simulink model "ssc_bridge_rectifier_rt"  (R2015b)
settings: Solver=ode3  StartTime=0.0  StopTime=0.05  FixedStep=Ts  MaxStep=0.001  RelTol=1e-3
PostLoadFcn:
  | Ts=100e-6;
InitFcn:
  | Ts=100e-6;
undefined symbols (not defined in the file): another_event_name, my_event_name
libraries: fl_lib x11, opal_lib x4, rtlab x3, nesl_utility x3
Description:
  | Full-Wave Bridge Rectifier
  | 
  | This is a model of a power supply that converts 120 volts AC to 12  volts DC. The
  | transformer has a turns ratio of 14, stepping the supply down to 8.6 volts rms, i.e.
  | 8.6*sqrt(2) = 12 volts pk-pk. The full-wave bridge rectifier plus capacitor combination
  | then converts this to DC. The resistor represents a typical load.
  | 
  | The model can be used to size the capacitor required for a specified load.  For a
  | given size of capacitor, as the load resistance is increased, the ripple on the DC
  | voltage increases. The model can also be used to drive an application circuit in
  | order to assess the effect of the ripple.
  | 
  | 
  | Copyright 2008 The MathWorks(TM), Inc.
settings Model: ExtModeAutoUpdateStatusClock=off  Creator=rhyde  LastModifiedBy=NesrineBradai
settings DataIOCC: SaveFormat=Array  SignalLoggingSaveFormat=ModelDataLogs  SaveOutput=off  SignalLogging=off  SaveTime=off
settings OptimizationCC: BlockReduction=off  OptimizeBlockIOStorage=off  BufferReuse=off  ExpressionFolding=off  ExpressionDepthLimit=2147483647  LocalBlockOutputs=off  InitFltsAndDblsToZero=on
settings DebuggingCC: SaveWithParameterizedLinksMsg=none  UnderspecifiedInitializationDetection=Classic  MergeDetectMultiDrivingBlocksExec=none  SignalResolutionControl=TryResolveAllWithWarning  SolverPrmCheckMsg=warning  FcnCallInpInsideContextMsg=EnableAllAsWarning  AllowSymbolicDim=on  StateNameClashWarn=warning
settings HardwareCC: ProdBitPerPointer=32  ProdLargestAtomicFloat=None  ProdIntDivRoundTo=Undefined  ProdEndianess=Unspecified  ProdWordSize=32  ProdHWDeviceType=32-bit Generic
settings GRTTargetCC: TargetFcnLib=ansi_tfl_tmw.mat  CombineOutputUpdateFcns=off  GRTInterface=on
settings ConfigComp: CovModelRefEnable=Off
settings SimscapeCC: SimscapeNormalizeSystem=off

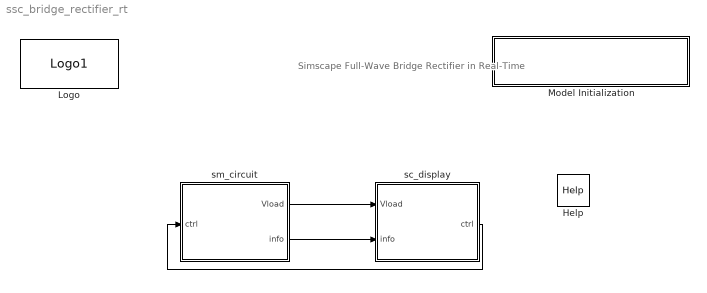
== system ssc_bridge_rectifier_rt ==
  note: Simscape Full-Wave Bridge Rectifier in Real-Time
  Help : opal_lib/Help  docfile=../../help/help.html
  Logo : opal_lib/Logo1  vide=[]
  Model Initialization : Subsystem  mask(Model Functions){InitFcnX=Ts=100e-6;, prel=off, posl=on, inif=on, strf=off}
      mask prompts: InitFcnX "Initialisation"; prel "Preload Function"; posl "PostLoad Function"; inif "InitFcn"; strf "StartFcn"
      mask init:
      | currentBlock = gcb;
      | root = bdroot(currentBlock);
      | 
      | if ~strcmp(get_param(root,'BlockDiagramType'),'library')
      |     if prel==1
      |         set_param(root, 'PreLoadFcn', InitFcnX);
      |     else
      |         set_param(root, 'PreLoadFcn', '');
      |     end
      |     if inif==1
      |         set_param(root, 'InitFcn', InitFcnX);
      |     else
      |         set_param(root, 'InitFcn', '');
      |     end
      |     if strf==1
      |         set_param(root, 'StartFcn', InitFcnX);
      |     else
      |         set_param(root, 'StartFcn', '');
      |     end
      |     if posl==1
      |         set_param(root, 'PostLoadFcn', InitFcnX);
      |     else
      |         set_param(root, 'PostLoadFcn', '');
      |     end
      | end
      | 
      | pos = get_param(currentBlock, 'Position');
      | width = pos(3) - pos(1); height = pos(4) - pos(2);
      | txt = [ upper(root) '\n' '- InitFcn. . . . . '  get_param(root, 'InitFcn') ];
      settings: CopyFcn=set_param(gcb,'LinkStatus','none')
      mask Display: text(5, height*0.5, txt, 'horizontalAlignment', 'left', 'verticalAlignment', 'middle') ;
  sc_display : Subsystem
  sm_circuit : Subsystem
  wires:
  sm_circuit/1(Vload) -> sc_display/1(Vload)
  sm_circuit/2(info) -> sc_display/2(info)
  sc_display/1(ctrl) -> sm_circuit/1(ctrl)

== system ssc_bridge_rectifier_rt/Model Initialization ==

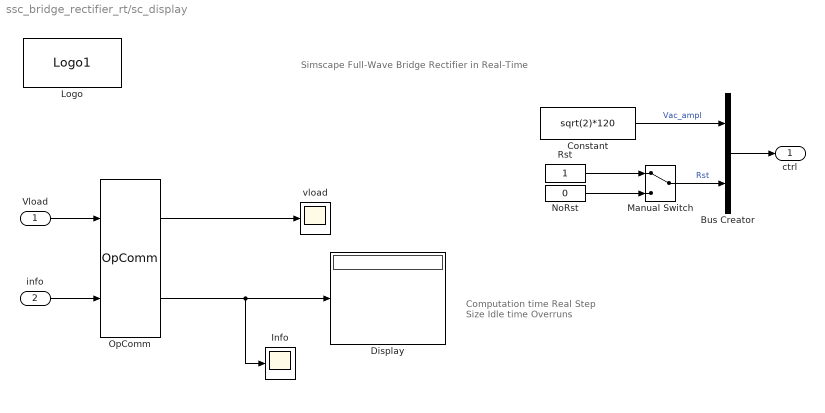
== system ssc_bridge_rectifier_rt/sc_display ==
  note: Computation time
      | Real Step Size
      | Idle time
      | Overruns
  note: Simscape Full-Wave Bridge Rectifier in Real-Time
  Vload : Inport
  info : Inport  Port=2
  Bus Creator : BusCreator  Inputs=2
  Constant : Constant  Value=sqrt(2)*120
  Display : Display
  Info : Scope
  Logo : opal_lib/Logo1  vide=[]
  Manual Switch : ManualSwitch
  NoRst : Constant  Value=0
  OpComm : rtlab/OpComm  nbport=2  groupe_acq=1  subsys_rate=0  st=0  Synchronization=on  Interpolation=on  Threshold=1.0  Missed_Data=off  Sim_Time=off  Samples=off  dynSigOut=off  from_console=0  warning_done=off  writeOpCommFile=off  Offset=off
  Rst : Constant
  vload : Scope
  ctrl : Outport
  wires:
  Vload/1 -> OpComm/1
  OpComm/1 -> vload/1
  info/1 -> OpComm/2
  OpComm/2 -> Info/1, Display/1
  Rst/1 -> Manual Switch/1
  NoRst/1 -> Manual Switch/2
  Bus Creator/1 -> ctrl/1
  Constant/1 -> Bus Creator/1  "Vac_ampl"
  Manual Switch/1 -> Bus Creator/2  "Rst"

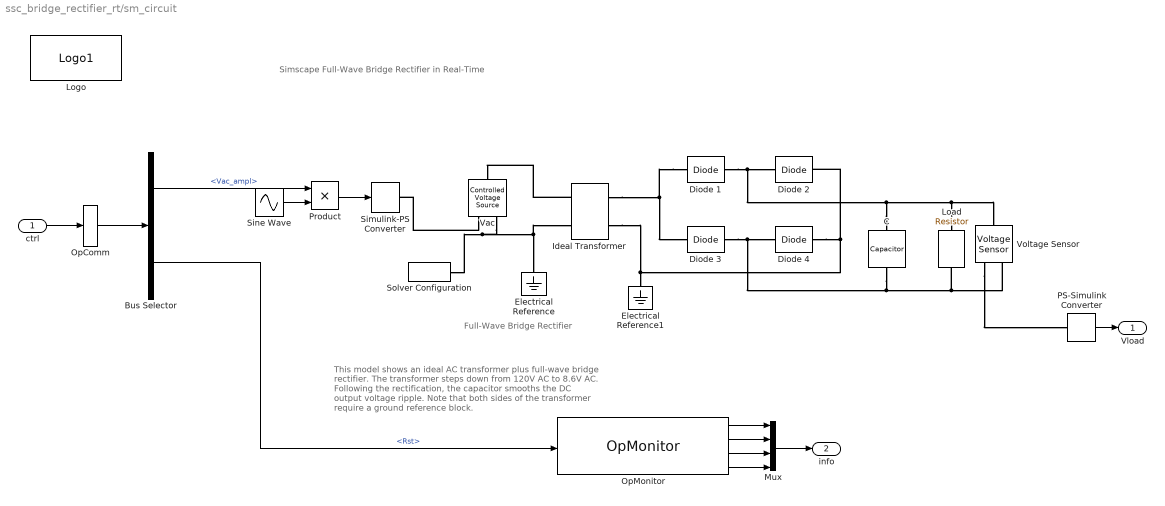
== system ssc_bridge_rectifier_rt/sm_circuit ==
  note: Full-Wave Bridge Rectifier
  note: This model shows an ideal AC transformer plus
      | full-wave bridge rectifier. The transformer steps
      | down from 120V AC to 8.6V AC. Following the rectification,
      | the capacitor smooths the DC output voltage ripple. Note
      | that both sides of the transformer require a ground
      | reference block.
  note: Simscape Full-Wave Bridge Rectifier in Real-Time
  ctrl : Inport
  Bus Selector : BusSelector  OutputSignals=Vac_ampl,Rst
  C : fl_lib/Electrical/Electrical Elements/Capacitor  c=470e-06 F  r=1e-06 Ohm  g=0 1/Ohm  i_specify=off  i_priority=High  i=0 A  i_nominal_specify=off  i_nominal_unit=A  i_nominal_value=1  v_specify=off  v_priority=High  v=0 V  v_nominal_specify=off  v_nominal_unit=V  v_nominal_value=1  vc_specify=on  vc_priority=High  vc=0 V  vc_nominal_specify=off  vc_nominal_unit=V  vc_nominal_value=1
  Diode {1..4} (4 alike) : fl_lib/Electrical/Electrical Elements/Diode  Vf=0.6 V  Ron=0.3 Ohm  Goff=1e-08 1/Ohm  i_specify=off  i_priority=High  i=0 A  i_nominal_specify=off  i_nominal_unit=A  i_nominal_value=1  v_specify=off  v_priority=High  v=0 V  v_nominal_specify=off  v_nominal_unit=V  v_nominal_value=1
  Electrical Reference : fl_lib/Electrical/Electrical Elements/Electrical Reference
  Electrical Reference1 : fl_lib/Electrical/Electrical Elements/Electrical Reference
  Ideal Transformer : fl_lib/Electrical/Electrical Elements/Ideal Transformer  n=14  i1_specify=off  i1_priority=High  i1=0 A  i1_nominal_specify=off  i1_nominal_unit=A  i1_nominal_value=1  v1_specify=off  v1_priority=High  v1=0 V  v1_nominal_specify=off  v1_nominal_unit=V  v1_nominal_value=1  i2_specify=off  i2_priority=High  i2=0 A  i2_nominal_specify=off  i2_nominal_unit=A  i2_nominal_value=1  v2_specify=off  v2_priority=High  v2=0 V  v2_nominal_specify=off  v2_nominal_unit=V  v2_nominal_value=1
  Load : fl_lib/Electrical/Electrical Elements/Resistor  R=100 Ohm  i_specify=off  i_priority=High  i=0 A  i_nominal_specify=off  i_nominal_unit=A  i_nominal_value=1  v_specify=off  v_priority=High  v=0 V  v_nominal_specify=off  v_nominal_unit=V  v_nominal_value=1
  Logo : opal_lib/Logo1  vide=[]
  Mux : Mux
  OpComm : rtlab/OpComm  nbport=1  groupe_acq=1  subsys_rate=0  st=0  Synchronization=on  Interpolation=on  Threshold=1.0  Missed_Data=off  Sim_Time=off  Samples=off  dynSigOut=off  from_console=1  warning_done=off  writeOpCommFile=off  Offset=off
  OpMonitor : rtlab/Monitoring/OpMonitor  compute_time=on  real_step=on  idle_time=on  nb_overruns=on  user_time=off  user_name=my_event_name,another_event_name
  PS-Simulink Converter : nesl_utility/PS-Simulink Converter  PhysicalDomain=network_engine_domain  SubClassName=ps_output  LeftPortType=input  RightPortType=output  PseudoPeriodic=off  Frequencies=[]  Unit=1  AffineConversion=off
  Product : Product  RndMeth=Zero
  Simulink-PS Converter : nesl_utility/Simulink-PS Converter  PhysicalDomain=network_engine_domain  SubClassName=ps_input  LeftPortType=input  RightPortType=output  PseudoPeriodic=off  Frequencies=[]  NoiseDistribution=none  NoiseParameters=[]  Unit=1  AffineConversion=off  FilteringAndDerivatives=zero  SimscapeFilterOrder=1  InputFilterTimeConstant=.001  UdotUserProvided=0
  Sine Wave : Sin  Frequency=2*pi*60  SampleTime=0
  Solver Configuration : nesl_utility/Solver Configuration  PhysicalDomain=network_engine_domain  SubClassName=solver  LeftPortType=input  RightPortType=generic  Tones=[]  Harmonics=[]  SimulateNoise=off  Profile=off  UseLocalSampling=off  EnableSwitchedLinearOptims=on  FrequencyDomain=off  UseCCode=off  RelTol=0.001  AbsTol=1e-06  MinStep=1e-09  ToWorkspace=off  RevertToSquareIcSolve=off  NumHomotopyIterations=100  PhasorMode=off  PhasorModeNumHarmonics=1  DoDC=off  ResidualTolerance=1e-9  UseLocalSolver=off  LocalSolverChoice=NE_BACKWARD_EULER_ADVANCER  LocalSolverSampleTime=.001  DoFixedCost=off  MaxNonlinIter=12  MaxModeIter=2  ComputeImpulses=off  ImpulseIterations=2  LinearAlgebra=Sparse  EquationFormulation=NE_TIME_EF  DelaysMemoryBudget=1024  AutomaticFiltering=on  FilteringTimeConstant=0.001  PartitionStorageMethod=AS_NEEDED  PartitionMemoryBudget=1024  PartitionMethod=FAST
  Vac : fl_lib/Electrical/Electrical Sources/Controlled Voltage Source
  Voltage Sensor : fl_lib/Electrical/Electrical Sensors/Voltage Sensor
  Vload : Outport
  info : Outport  Port=2
  wires:
  PS-Simulink Converter/1 -> Vload/1
  Bus Selector/2 -> OpMonitor/1  "<Rst>"
  OpMonitor/1 -> Mux/1
  OpMonitor/2 -> Mux/2
  OpMonitor/3 -> Mux/3
  OpMonitor/4 -> Mux/4
  Mux/1 -> info/1
  ctrl/1 -> OpComm/1
  Sine Wave/1 -> Product/2
  Product/1 -> Simulink-PS Converter/1
  OpComm/1 -> Bus Selector/1
  Bus Selector/1 -> Product/1  "<Vac_ampl>"
  connections:
  Ideal Transformer/LConn1 -- Vac/LConn1
  Vac/RConn2 -- Solver Configuration/RConn1 -- Electrical Reference/LConn1 -- Ideal Transformer/LConn2
  C/LConn1 -- Load/LConn1 -- Voltage Sensor/LConn1 -- Diode 2/RConn1 -- Diode 1/RConn1
  C/RConn1 -- Load/RConn1 -- Voltage Sensor/RConn2 -- Diode 4/LConn1 -- Diode 3/LConn1
  Diode 1/LConn1 -- Diode 3/RConn1 -- Ideal Transformer/RConn1
  Diode 2/LConn1 -- Diode 4/RConn1 -- Electrical Reference1/LConn1 -- Ideal Transformer/RConn2
  Voltage Sensor/RConn1 -- PS-Simulink Converter/LConn1
  Vac/RConn1 -- Simulink-PS Converter/RConn1
